simulink model "HVDCMMCInterconnection"  (R2023b)
settings: Solver=FixedStepDiscrete  StartTime=0.0  StopTime=10  FixedStep=Ts_Power  RelTol=1e-4
PreLoadFcn:
  | HVDCMMCInterconnectionParam
StartFcn:
  | tic
StopFcn:
  | toc
values from neighbouring files (symbols this model uses):
  C_PM = 1.758e-3    (= 0.001758)    [HVDCMMCInterconnectionParam.m]
  Cg = 50e-9    (= 5e-08)    [HVDCMMCInterconnectionParam.m]
  D_R = 0.001    [HVDCMMCInterconnectionParam.m]
  D_Rs = 1e8    (= 100000000)    [HVDCMMCInterconnectionParam.m]
  D_Vf = 0    [HVDCMMCInterconnectionParam.m]
  Fnom = 50    [HVDCMMCInterconnectionParam.m]
  HRM = 2    [HVDCMMCInterconnectionParam.m]
  Ki_Ireg = 6    [HVDCMMCInterconnectionParam.m]
  Ki_Preg = 1.0    (= 1)    [HVDCMMCInterconnectionParam.m]
  Ki_Qreg = 1.0    (= 1)    [HVDCMMCInterconnectionParam.m]
  Ki_VDCreg = 100    [HVDCMMCInterconnectionParam.m]
  Kp_Ireg = 0.6    [HVDCMMCInterconnectionParam.m]
  Kp_Preg = 0.5/3    (= 0.166666666667)    [HVDCMMCInterconnectionParam.m]
  Kp_Qreg = 0.5/3    (= 0.166666666667)    [HVDCMMCInterconnectionParam.m]
  Kp_VDCreg = 4    [HVDCMMCInterconnectionParam.m]
  L_cable = 15e-3    (= 0.015)    [HVDCMMCInterconnectionParam.m]
  Larm = Larm_pu*(Zb_ac/(2*pi*Fnom))    [HVDCMMCInterconnectionParam.m]
  Lff = Larm_pu/2    (= 0.075)    [HVDCMMCInterconnectionParam.m]
  Limits_Ireg = [ 2.0  -2.0]    [HVDCMMCInterconnectionParam.m]
  Limits_Preg = [ 1.2, 0.8 ]    [HVDCMMCInterconnectionParam.m]
  Limits_Qreg = [ 0.25, -0.25 ]    [HVDCMMCInterconnectionParam.m]
  Limits_VDCreg = [ 2.0  -2.0]    [HVDCMMCInterconnectionParam.m]
  Lxfo = 0.12    [HVDCMMCInterconnectionParam.m]
  Nb_PM = 36    [HVDCMMCInterconnectionParam.m]
  Pnom = 1000e6    (= 1000000000)    [HVDCMMCInterconnectionParam.m]
  R_cable = 0.5    [HVDCMMCInterconnectionParam.m]
  R_startup = 400    [HVDCMMCInterconnectionParam.m]
  Rarm = Rarm_pu*Zb_ac    [HVDCMMCInterconnectionParam.m]
  Rff = Rarm_pu/2    (= 0.00075)    [HVDCMMCInterconnectionParam.m]
  Rg = 100    [HVDCMMCInterconnectionParam.m]
  Rxfo = 0.003    [HVDCMMCInterconnectionParam.m]
  Slope_Pref = 0.5    [HVDCMMCInterconnectionParam.m]
  Slope_Qref = 0.5    [HVDCMMCInterconnectionParam.m]
  Slope_Vdc_ref = Vnom_dc/5    (= 128000)    [HVDCMMCInterconnectionParam.m]
  Tbrk1_On = 0.1    [HVDCMMCInterconnectionParam.m]
  Tbrk2_On = 1.0    (= 1)    [HVDCMMCInterconnectionParam.m]
  Tdeblock = 1.5    [HVDCMMCInterconnectionParam.m]
  Tfault = 9999    [HVDCMMCInterconnectionParam.m]
  Ton_Converter2 = 4    [HVDCMMCInterconnectionParam.m]
  Ton_PQreg = 4    [HVDCMMCInterconnectionParam.m]
  Ton_VDCreg = 1.5    [HVDCMMCInterconnectionParam.m]
  Ts = Ts_Control    (= 4e-05)    [HVDCMMCInterconnectionParam.m]    (also in power_circ2ss_sps_calc.m = 1e-06)
  Ts_Control = 40e-6    (= 4e-05)    [HVDCMMCInterconnectionParam.m]
  Ts_Power = 20e-6    (= 2e-05)    [HVDCMMCInterconnectionParam.m]
  Vb_ac = sqrt(2/3)*Vnom_sec    [HVDCMMCInterconnectionParam.m]
  Vb_dc = Vnom_dc    (= 640000)    [HVDCMMCInterconnectionParam.m]
  Vc0_PM = 0    [HVDCMMCInterconnectionParam.m]
  Vnom_dc = 640e3    (= 640000)    [HVDCMMCInterconnectionParam.m]
  Vnom_prim = 400e3    (= 400000)    [HVDCMMCInterconnectionParam.m]
  Vnom_sec = 333e3    (= 333000)    [HVDCMMCInterconnectionParam.m]
  w = 2*pi*Fnom    (= 314.159265359)    [HVDCMMCInterconnectionParam.m]
undefined symbols (not defined in the file or in its folder): ACDC, ACDC3, DiscIntNeverNeededParam, gcbh, Pcc, S, sps_AC, sps_rtmsupport
libraries: simulink x61, spsControlledVoltageSourceLib x56, spsCurrentMeasurementLib x56, spsDiodeLib x40, spsSeriesRLCBranchLib x32, spsVoltageMeasurementLib x20, powerlib_extras x9, spsHalfBridgeMMCmodel x8, spsGroundLib x7, spsSecondOrderFilterLib x6, spsabctodq0Lib x6, spsMeanLib x3
(part 4 of 11)

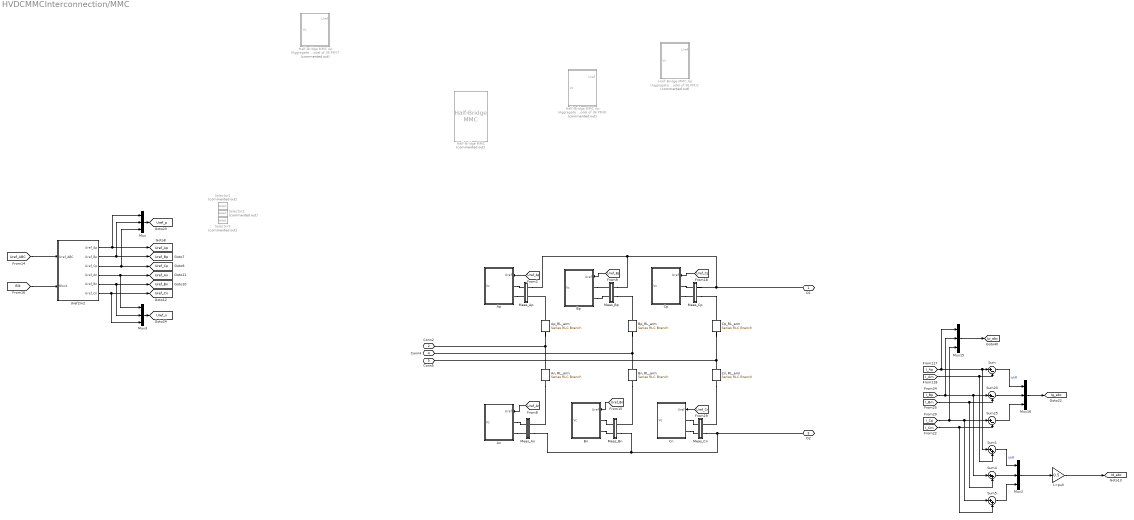
== system HVDCMMCInterconnection/MMC ==
  An : Subsystem  DialogController=POWERSYS.PowerSysDialog  LoadFcn=sps_rtmsupport('LoadFcn',gcbh);  StartFcn=sps_rtmsupport('StartFcn',gcbh);  StopFcn=sps_rtmsupport('StopFcn',gcbh);  mask(Half-Bridge MMC){ModelType=Aggregate model, n=36, C=C_PM, Vc_Initial=Vc0_PM, Ron=1e-3, Rs=1e6, Cs=inf, Ron_Diode=1e-3, Rs_Diode=1e6, Cs_Diode=inf, Vf_Diode=1e-3, Rs_CurrentSource=inf, Ts=Ts_Power}
      mask prompts: ModelType "Model type:"; n "Number of power modules"; C "Capacitor value (F)"; Vc_Initial "Capacitor initial voltage (V):"; Ron "Device on-state resistance (Ohms)"; Rs "Snubber resistance (Ohms)"; Cs "Snubber capacitance (F)"; Ron_Diode "Diode on-state resistance (Ohms)"; Rs_Diode "Diode snubber resistance (Ohms)"; Cs_Diode "Diode snubber capacitance (F)"; Vf_Diode "Diode forward voltage (V)"; Rs_CurrentSource "Current source snubber resistance (Ohms)"; Ts "Sample time (s):"
      mask help: Implements a half-bridge modular multilevel converter. The converter consists of multiple series-connected power modules. Each power module consists of one half-bridge and one capacitor on the DC side.
      mask init:
      | % block=gcb;
      | % [WantBlockChoice,Index1,MT,SPID] = powericon('FullBridgeMMCInit', block, ModelType, n, Ts, 2);
      | % powericon('SetInternalModels','set',block,WantBlockChoice);
      settings: LibrarySourceBlock=spsHalfBridgeMMCLib/Half-Bridge MMC  CopyFcn=sps_rtmsupport('CopyFcn',gcbh);  DeleteFcn=sps_rtmsupport('DeleteFcn',gcbh);  UndoDeleteFcn=sps_rtmsupport('UndoDeleteFcn',gcbh);  ModelCloseFcn=sps_rtmsupport('ModelCloseFcn',gcbh);  PreSaveFcn=sps_rtmsupport('PreSaveFcn',gcbh);  PostSaveFcn=sps_rtmsupport('PostSaveFcn',gcbh);  NameChangeFcn=sps_rtmsupport('NameChangeFcn',gcbh);  PreCopyFcn=sps_rtmsupport('PreCopyFcn',gcbh);  OpenFcn=sps_rtmsupport('OpenFcn',gcbh, [1]);  CloseFcn=sps_rtmsupport('CloseFcn',gcbh);  PreDeleteFcn=sps_rtmsupport('PreDeleteFcn',gcbh);
      mask Help: helpview(psbhelp);
      mask TypeOptions ModelType: Switching devices | Switching function | Average model (Uref-controlled) | Aggregate model
      mask Callback ModelType: powericon('FullBridgeMMCCback',gcb)
      mask Display:
      | x1=-0.04;
      | plot([0.5 0.80]+x1,[0.95 0.95])
      | plot([0.5 0.5]+x1,[0.95,0.80])
      | plot([0.5 0.38]+x1,[0.80 0.74])
      | plot([0.38 0.38]+x1,[0.80 0.62])
      | plot([0.38 0.5]+x1,[0.68 0.62])
      | plot([0.5 0.5]+x1,[0.62 0.52])
      | plot([0.45 0.5 0.43]+x1,[0.68 0.62 0.60])
      | %
      | y1=0.40;
      | plot([0.5 0.5]+x1,[0.95,0.80]-y1)
      | plot([0.5 0.38]+x1,[0.80 0.74]-y1)
      | plot([0.38 0.38]+x1,[0.80 0.62]-y1)
      | plot([0.38 0.5]+x1,[0.68 0.62]-y1)
      | plot([0.5 0.5]+x1,[0.62 0.52]-y1)
      | plot([0.45 0.5 0.43]+x1,[0.68 0.62 0.60]-y1)
      | plot([0.5 0.5]+x1,[0.2,0.10])
      | plot([0.5 0.80]+x1,[0.1 0.1])
      | %
      | plot([0.5 0.6]+x1,[0.84 0.84])
      | plot([0.6 0.6]+x1,[0.84 0.74])
      | plot([0.6 0.56]+x1,[0.74 0.69])
      | plot([0.6 0.64]+x1,[0.74 0.69])
      | plot([0.56 0.64]+x1,[0.69 0.69])
      | plot([0.6 0.6]+x1,[0.69 0.57])
      | plot([0.5 0.6]+x1,[0.57 0.57])
      | plot([0.55 0.65]+x1,[0.74 0.74])
      | %
      | y2=0.4;
      | plot([0.5 0.6]+x1,[0.84 0.84]-y2)
      | plot([0.6 0.6]+x1,[0.84 0.74]-y2)
      | plot([0.6 0.56]+x1,[0.74 0.69]-y2)
      | plot([0.6 0.64]+x1,[0.74 0.69]-y2)
      | plot([0.56 0.64]+x1,[0.69 0.69]-y2)
      | plot([0.6 0.6]+x1,[0.69 0.57]-y2)
      | plot([0.5 0.6]+x1,[0.57 0.57]-y2)
      | plot([0.55 0.65]+x1,[0.74 0.74]-y2)
      | %
      | plot([0.5 0.23]+x1,[0.5 0.5])
      | plot([0.23 0.23]+x1,[0.5 0.53])
      | plot([0.23 0.23]+x1,[0.55 0.58])
      | plot([0.23 0.23]+x1,[0.61 0.64])
      | %
      | plot([0.5 0.23]+x1,[0.1 0.1])
      | plot([0.23 0.23]+x1,[0.1 0.06])
      | plot([0.23 0.23]+x1,[0.04 0.01])
      | %
      | plot([0.34 0.34]+x1,[0.65 0.75])
      | plot([0.28 0.34]+x1,[0.7 0.7])
      | %
      | plot([0.34 0.34]+x1,[0.65 0.75]-y2)
      | plot([0.28 0.34]+x1,[0.7 0.7]-y2)
      | %
      | % Capacitor
      | plot([0.8 0.8]+x1,[0.51 0.95])
      | plot([0.72 0.88]+x1,[0.51 0.51])
      | plot([0.72 0.88]+x1,[0.51 0.51]-0.04)
      | plot([0.8 0.8]+x1,[0.47 0.1])
      | 
      | color('blue')
      | % switch lower(ModelType)
      | %     case 'average model (uref-controlled)'
      | %         port_label('input',1,'Uref')
      | %     case 'aggregate model'
      | %         port_label('input',1,'Uref')
      | %     otherwise
      | %         port_label('input',1,'Uref')
      | % end
      | port_label('output',1,'m')
  An_RL_arm : spsSeriesRLCBranchLib/Series RLC Branch  LConnTagsString=__new0  RConnTagsString=__new0  BranchType=RL  Resistance=Rarm  Inductance=Larm  SetiL0=off  InitialCurrent=0  Capacitance=1e-6  Setx0=off  InitialVoltage=0  Measurements=None
  Ap : Subsystem  DialogController=POWERSYS.PowerSysDialog  LoadFcn=sps_rtmsupport('LoadFcn',gcbh);  StartFcn=sps_rtmsupport('StartFcn',gcbh);  StopFcn=sps_rtmsupport('StopFcn',gcbh);  mask(Half-Bridge MMC){ModelType=Aggregate model, n=36, C=C_PM, Vc_Initial=Vc0_PM, Ron=1e-3, Rs=1e6, Cs=inf, Ron_Diode=1e-3, Rs_Diode=1e6, Cs_Diode=inf, Vf_Diode=1e-3, Rs_CurrentSource=inf, Ts=Ts_Power}
      mask prompts: ModelType "Model type:"; n "Number of power modules"; C "Capacitor value (F)"; Vc_Initial "Capacitor initial voltage (V):"; Ron "Device on-state resistance (Ohms)"; Rs "Snubber resistance (Ohms)"; Cs "Snubber capacitance (F)"; Ron_Diode "Diode on-state resistance (Ohms)"; Rs_Diode "Diode snubber resistance (Ohms)"; Cs_Diode "Diode snubber capacitance (F)"; Vf_Diode "Diode forward voltage (V)"; Rs_CurrentSource "Current source snubber resistance (Ohms)"; Ts "Sample time (s):"
      mask help: Implements a half-bridge modular multilevel converter. The converter consists of multiple series-connected power modules. Each power module consists of one half-bridge and one capacitor on the DC side.
      mask init:
      | % block=gcb;
      | % [WantBlockChoice,Index1,MT,SPID] = powericon('FullBridgeMMCInit', block, ModelType, n, Ts, 2);
      | % powericon('SetInternalModels','set',block,WantBlockChoice);
      settings: LibrarySourceBlock=spsHalfBridgeMMCLib/Half-Bridge MMC  CopyFcn=sps_rtmsupport('CopyFcn',gcbh);  DeleteFcn=sps_rtmsupport('DeleteFcn',gcbh);  UndoDeleteFcn=sps_rtmsupport('UndoDeleteFcn',gcbh);  ModelCloseFcn=sps_rtmsupport('ModelCloseFcn',gcbh);  PreSaveFcn=sps_rtmsupport('PreSaveFcn',gcbh);  PostSaveFcn=sps_rtmsupport('PostSaveFcn',gcbh);  NameChangeFcn=sps_rtmsupport('NameChangeFcn',gcbh);  PreCopyFcn=sps_rtmsupport('PreCopyFcn',gcbh);  OpenFcn=sps_rtmsupport('OpenFcn',gcbh, [1]);  CloseFcn=sps_rtmsupport('CloseFcn',gcbh);  PreDeleteFcn=sps_rtmsupport('PreDeleteFcn',gcbh);
      mask Help: helpview(psbhelp);
      mask TypeOptions ModelType: Switching devices | Switching function | Average model (Uref-controlled) | Aggregate model
      mask Callback ModelType: powericon('FullBridgeMMCCback',gcb)
      mask Display:
      | x1=-0.04;
      | plot([0.5 0.80]+x1,[0.95 0.95])
      | plot([0.5 0.5]+x1,[0.95,0.80])
      | plot([0.5 0.38]+x1,[0.80 0.74])
      | plot([0.38 0.38]+x1,[0.80 0.62])
      | plot([0.38 0.5]+x1,[0.68 0.62])
      | plot([0.5 0.5]+x1,[0.62 0.52])
      | plot([0.45 0.5 0.43]+x1,[0.68 0.62 0.60])
      | %
      | y1=0.40;
      | plot([0.5 0.5]+x1,[0.95,0.80]-y1)
      | plot([0.5 0.38]+x1,[0.80 0.74]-y1)
      | plot([0.38 0.38]+x1,[0.80 0.62]-y1)
      | plot([0.38 0.5]+x1,[0.68 0.62]-y1)
      | plot([0.5 0.5]+x1,[0.62 0.52]-y1)
      | plot([0.45 0.5 0.43]+x1,[0.68 0.62 0.60]-y1)
      | plot([0.5 0.5]+x1,[0.2,0.10])
      | plot([0.5 0.80]+x1,[0.1 0.1])
      | %
      | plot([0.5 0.6]+x1,[0.84 0.84])
      | plot([0.6 0.6]+x1,[0.84 0.74])
      | plot([0.6 0.56]+x1,[0.74 0.69])
      | plot([0.6 0.64]+x1,[0.74 0.69])
      | plot([0.56 0.64]+x1,[0.69 0.69])
      | plot([0.6 0.6]+x1,[0.69 0.57])
      | plot([0.5 0.6]+x1,[0.57 0.57])
      | plot([0.55 0.65]+x1,[0.74 0.74])
      | %
      | y2=0.4;
      | plot([0.5 0.6]+x1,[0.84 0.84]-y2)
      | plot([0.6 0.6]+x1,[0.84 0.74]-y2)
      | plot([0.6 0.56]+x1,[0.74 0.69]-y2)
      | plot([0.6 0.64]+x1,[0.74 0.69]-y2)
      | plot([0.56 0.64]+x1,[0.69 0.69]-y2)
      | plot([0.6 0.6]+x1,[0.69 0.57]-y2)
      | plot([0.5 0.6]+x1,[0.57 0.57]-y2)
      | plot([0.55 0.65]+x1,[0.74 0.74]-y2)
      | %
      | plot([0.5 0.23]+x1,[0.5 0.5])
      | plot([0.23 0.23]+x1,[0.5 0.53])
      | plot([0.23 0.23]+x1,[0.55 0.58])
      | plot([0.23 0.23]+x1,[0.61 0.64])
      | %
      | plot([0.5 0.23]+x1,[0.1 0.1])
      | plot([0.23 0.23]+x1,[0.1 0.06])
      | plot([0.23 0.23]+x1,[0.04 0.01])
      | %
      | plot([0.34 0.34]+x1,[0.65 0.75])
      | plot([0.28 0.34]+x1,[0.7 0.7])
      | %
      | plot([0.34 0.34]+x1,[0.65 0.75]-y2)
      | plot([0.28 0.34]+x1,[0.7 0.7]-y2)
      | %
      | % Capacitor
      | plot([0.8 0.8]+x1,[0.51 0.95])
      | plot([0.72 0.88]+x1,[0.51 0.51])
      | plot([0.72 0.88]+x1,[0.51 0.51]-0.04)
      | plot([0.8 0.8]+x1,[0.47 0.1])
      | 
      | color('blue')
      | % switch lower(ModelType)
      | %     case 'average model (uref-controlled)'
      | %         port_label('input',1,'Uref')
      | %     case 'aggregate model'
      | %         port_label('input',1,'Uref')
      | %     otherwise
      | %         port_label('input',1,'Uref')
      | % end
      | port_label('output',1,'m')
  Ap_RL_arm : spsSeriesRLCBranchLib/Series RLC Branch  LConnTagsString=__new0  RConnTagsString=__new0  BranchType=RL  Resistance=Rarm  Inductance=Larm  SetiL0=off  InitialCurrent=0  Capacitance=1e-6  Setx0=off  InitialVoltage=0  Measurements=None
  Bn : Subsystem  DialogController=POWERSYS.PowerSysDialog  LoadFcn=sps_rtmsupport('LoadFcn',gcbh);  StartFcn=sps_rtmsupport('StartFcn',gcbh);  StopFcn=sps_rtmsupport('StopFcn',gcbh);  mask(Half-Bridge MMC){ModelType=Aggregate model, n=36, C=C_PM, Vc_Initial=Vc0_PM, Ron=1e-3, Rs=1e6, Cs=inf, Ron_Diode=1e-3, Rs_Diode=1e6, Cs_Diode=inf, Vf_Diode=1e-3, Rs_CurrentSource=inf, Ts=Ts_Power}
      mask prompts: ModelType "Model type:"; n "Number of power modules"; C "Capacitor value (F)"; Vc_Initial "Capacitor initial voltage (V):"; Ron "Device on-state resistance (Ohms)"; Rs "Snubber resistance (Ohms)"; Cs "Snubber capacitance (F)"; Ron_Diode "Diode on-state resistance (Ohms)"; Rs_Diode "Diode snubber resistance (Ohms)"; Cs_Diode "Diode snubber capacitance (F)"; Vf_Diode "Diode forward voltage (V)"; Rs_CurrentSource "Current source snubber resistance (Ohms)"; Ts "Sample time (s):"
      mask help: Implements a half-bridge modular multilevel converter. The converter consists of multiple series-connected power modules. Each power module consists of one half-bridge and one capacitor on the DC side.
      mask init:
      | % block=gcb;
      | % [WantBlockChoice,Index1,MT,SPID] = powericon('FullBridgeMMCInit', block, ModelType, n, Ts, 2);
      | % powericon('SetInternalModels','set',block,WantBlockChoice);
      settings: LibrarySourceBlock=spsHalfBridgeMMCLib/Half-Bridge MMC  CopyFcn=sps_rtmsupport('CopyFcn',gcbh);  DeleteFcn=sps_rtmsupport('DeleteFcn',gcbh);  UndoDeleteFcn=sps_rtmsupport('UndoDeleteFcn',gcbh);  ModelCloseFcn=sps_rtmsupport('ModelCloseFcn',gcbh);  PreSaveFcn=sps_rtmsupport('PreSaveFcn',gcbh);  PostSaveFcn=sps_rtmsupport('PostSaveFcn',gcbh);  NameChangeFcn=sps_rtmsupport('NameChangeFcn',gcbh);  PreCopyFcn=sps_rtmsupport('PreCopyFcn',gcbh);  OpenFcn=sps_rtmsupport('OpenFcn',gcbh, [1]);  CloseFcn=sps_rtmsupport('CloseFcn',gcbh);  PreDeleteFcn=sps_rtmsupport('PreDeleteFcn',gcbh);
      mask Help: helpview(psbhelp);
      mask TypeOptions ModelType: Switching devices | Switching function | Average model (Uref-controlled) | Aggregate model
      mask Callback ModelType: powericon('FullBridgeMMCCback',gcb)
      mask Display:
      | x1=-0.04;
      | plot([0.5 0.80]+x1,[0.95 0.95])
      | plot([0.5 0.5]+x1,[0.95,0.80])
      | plot([0.5 0.38]+x1,[0.80 0.74])
      | plot([0.38 0.38]+x1,[0.80 0.62])
      | plot([0.38 0.5]+x1,[0.68 0.62])
      | plot([0.5 0.5]+x1,[0.62 0.52])
      | plot([0.45 0.5 0.43]+x1,[0.68 0.62 0.60])
      | %
      | y1=0.40;
      | plot([0.5 0.5]+x1,[0.95,0.80]-y1)
      | plot([0.5 0.38]+x1,[0.80 0.74]-y1)
      | plot([0.38 0.38]+x1,[0.80 0.62]-y1)
      | plot([0.38 0.5]+x1,[0.68 0.62]-y1)
      | plot([0.5 0.5]+x1,[0.62 0.52]-y1)
      | plot([0.45 0.5 0.43]+x1,[0.68 0.62 0.60]-y1)
      | plot([0.5 0.5]+x1,[0.2,0.10])
      | plot([0.5 0.80]+x1,[0.1 0.1])
      | %
      | plot([0.5 0.6]+x1,[0.84 0.84])
      | plot([0.6 0.6]+x1,[0.84 0.74])
      | plot([0.6 0.56]+x1,[0.74 0.69])
      | plot([0.6 0.64]+x1,[0.74 0.69])
      | plot([0.56 0.64]+x1,[0.69 0.69])
      | plot([0.6 0.6]+x1,[0.69 0.57])
      | plot([0.5 0.6]+x1,[0.57 0.57])
      | plot([0.55 0.65]+x1,[0.74 0.74])
      | %
      | y2=0.4;
      | plot([0.5 0.6]+x1,[0.84 0.84]-y2)
      | plot([0.6 0.6]+x1,[0.84 0.74]-y2)
      | plot([0.6 0.56]+x1,[0.74 0.69]-y2)
      | plot([0.6 0.64]+x1,[0.74 0.69]-y2)
      | plot([0.56 0.64]+x1,[0.69 0.69]-y2)
      | plot([0.6 0.6]+x1,[0.69 0.57]-y2)
      | plot([0.5 0.6]+x1,[0.57 0.57]-y2)
      | plot([0.55 0.65]+x1,[0.74 0.74]-y2)
      | %
      | plot([0.5 0.23]+x1,[0.5 0.5])
      | plot([0.23 0.23]+x1,[0.5 0.53])
      | plot([0.23 0.23]+x1,[0.55 0.58])
      | plot([0.23 0.23]+x1,[0.61 0.64])
      | %
      | plot([0.5 0.23]+x1,[0.1 0.1])
      | plot([0.23 0.23]+x1,[0.1 0.06])
      | plot([0.23 0.23]+x1,[0.04 0.01])
      | %
      | plot([0.34 0.34]+x1,[0.65 0.75])
      | plot([0.28 0.34]+x1,[0.7 0.7])
      | %
      | plot([0.34 0.34]+x1,[0.65 0.75]-y2)
      | plot([0.28 0.34]+x1,[0.7 0.7]-y2)
      | %
      | % Capacitor
      | plot([0.8 0.8]+x1,[0.51 0.95])
      | plot([0.72 0.88]+x1,[0.51 0.51])
      | plot([0.72 0.88]+x1,[0.51 0.51]-0.04)
      | plot([0.8 0.8]+x1,[0.47 0.1])
      | 
      | color('blue')
      | % switch lower(ModelType)
      | %     case 'average model (uref-controlled)'
      | %         port_label('input',1,'Uref')
      | %     case 'aggregate model'
      | %         port_label('input',1,'Uref')
      | %     otherwise
      | %         port_label('input',1,'Uref')
      | % end
      | port_label('output',1,'m')
  Bn_RL_arm : spsSeriesRLCBranchLib/Series RLC Branch  LConnTagsString=__new0  RConnTagsString=__new0  BranchType=RL  Resistance=Rarm  Inductance=Larm  SetiL0=off  InitialCurrent=0  Capacitance=1e-6  Setx0=off  InitialVoltage=0  Measurements=None
  Bp : Subsystem  DialogController=POWERSYS.PowerSysDialog  LoadFcn=sps_rtmsupport('LoadFcn',gcbh);  StartFcn=sps_rtmsupport('StartFcn',gcbh);  StopFcn=sps_rtmsupport('StopFcn',gcbh);  mask(Half-Bridge MMC){ModelType=Aggregate model, n=36, C=C_PM, Vc_Initial=Vc0_PM, Ron=1e-3, Rs=1e6, Cs=inf, Ron_Diode=1e-3, Rs_Diode=1e6, Cs_Diode=inf, Vf_Diode=1e-3, Rs_CurrentSource=inf, Ts=Ts_Power}
      mask prompts: ModelType "Model type:"; n "Number of power modules"; C "Capacitor value (F)"; Vc_Initial "Capacitor initial voltage (V):"; Ron "Device on-state resistance (Ohms)"; Rs "Snubber resistance (Ohms)"; Cs "Snubber capacitance (F)"; Ron_Diode "Diode on-state resistance (Ohms)"; Rs_Diode "Diode snubber resistance (Ohms)"; Cs_Diode "Diode snubber capacitance (F)"; Vf_Diode "Diode forward voltage (V)"; Rs_CurrentSource "Current source snubber resistance (Ohms)"; Ts "Sample time (s):"
      mask help: Implements a half-bridge modular multilevel converter. The converter consists of multiple series-connected power modules. Each power module consists of one half-bridge and one capacitor on the DC side.
      mask init:
      | % block=gcb;
      | % [WantBlockChoice,Index1,MT,SPID] = powericon('FullBridgeMMCInit', block, ModelType, n, Ts, 2);
      | % powericon('SetInternalModels','set',block,WantBlockChoice);
      settings: LibrarySourceBlock=spsHalfBridgeMMCLib/Half-Bridge MMC  CopyFcn=sps_rtmsupport('CopyFcn',gcbh);  DeleteFcn=sps_rtmsupport('DeleteFcn',gcbh);  UndoDeleteFcn=sps_rtmsupport('UndoDeleteFcn',gcbh);  ModelCloseFcn=sps_rtmsupport('ModelCloseFcn',gcbh);  PreSaveFcn=sps_rtmsupport('PreSaveFcn',gcbh);  PostSaveFcn=sps_rtmsupport('PostSaveFcn',gcbh);  NameChangeFcn=sps_rtmsupport('NameChangeFcn',gcbh);  PreCopyFcn=sps_rtmsupport('PreCopyFcn',gcbh);  OpenFcn=sps_rtmsupport('OpenFcn',gcbh, [1]);  CloseFcn=sps_rtmsupport('CloseFcn',gcbh);  PreDeleteFcn=sps_rtmsupport('PreDeleteFcn',gcbh);
      mask Help: helpview(psbhelp);
      mask TypeOptions ModelType: Switching devices | Switching function | Average model (Uref-controlled) | Aggregate model
      mask Callback ModelType: powericon('FullBridgeMMCCback',gcb)
      mask Display:
      | x1=-0.04;
      | plot([0.5 0.80]+x1,[0.95 0.95])
      | plot([0.5 0.5]+x1,[0.95,0.80])
      | plot([0.5 0.38]+x1,[0.80 0.74])
      | plot([0.38 0.38]+x1,[0.80 0.62])
      | plot([0.38 0.5]+x1,[0.68 0.62])
      | plot([0.5 0.5]+x1,[0.62 0.52])
      | plot([0.45 0.5 0.43]+x1,[0.68 0.62 0.60])
      | %
      | y1=0.40;
      | plot([0.5 0.5]+x1,[0.95,0.80]-y1)
      | plot([0.5 0.38]+x1,[0.80 0.74]-y1)
      | plot([0.38 0.38]+x1,[0.80 0.62]-y1)
      | plot([0.38 0.5]+x1,[0.68 0.62]-y1)
      | plot([0.5 0.5]+x1,[0.62 0.52]-y1)
      | plot([0.45 0.5 0.43]+x1,[0.68 0.62 0.60]-y1)
      | plot([0.5 0.5]+x1,[0.2,0.10])
      | plot([0.5 0.80]+x1,[0.1 0.1])
      | %
      | plot([0.5 0.6]+x1,[0.84 0.84])
      | plot([0.6 0.6]+x1,[0.84 0.74])
      | plot([0.6 0.56]+x1,[0.74 0.69])
      | plot([0.6 0.64]+x1,[0.74 0.69])
      | plot([0.56 0.64]+x1,[0.69 0.69])
      | plot([0.6 0.6]+x1,[0.69 0.57])
      | plot([0.5 0.6]+x1,[0.57 0.57])
      | plot([0.55 0.65]+x1,[0.74 0.74])
      | %
      | y2=0.4;
      | plot([0.5 0.6]+x1,[0.84 0.84]-y2)
      | plot([0.6 0.6]+x1,[0.84 0.74]-y2)
      | plot([0.6 0.56]+x1,[0.74 0.69]-y2)
      | plot([0.6 0.64]+x1,[0.74 0.69]-y2)
      | plot([0.56 0.64]+x1,[0.69 0.69]-y2)
      | plot([0.6 0.6]+x1,[0.69 0.57]-y2)
      | plot([0.5 0.6]+x1,[0.57 0.57]-y2)
      | plot([0.55 0.65]+x1,[0.74 0.74]-y2)
      | %
      | plot([0.5 0.23]+x1,[0.5 0.5])
      | plot([0.23 0.23]+x1,[0.5 0.53])
      | plot([0.23 0.23]+x1,[0.55 0.58])
      | plot([0.23 0.23]+x1,[0.61 0.64])
      | %
      | plot([0.5 0.23]+x1,[0.1 0.1])
      | plot([0.23 0.23]+x1,[0.1 0.06])
      | plot([0.23 0.23]+x1,[0.04 0.01])
      | %
      | plot([0.34 0.34]+x1,[0.65 0.75])
      | plot([0.28 0.34]+x1,[0.7 0.7])
      | %
      | plot([0.34 0.34]+x1,[0.65 0.75]-y2)
      | plot([0.28 0.34]+x1,[0.7 0.7]-y2)
      | %
      | % Capacitor
      | plot([0.8 0.8]+x1,[0.51 0.95])
      | plot([0.72 0.88]+x1,[0.51 0.51])
      | plot([0.72 0.88]+x1,[0.51 0.51]-0.04)
      | plot([0.8 0.8]+x1,[0.47 0.1])
      | 
      | color('blue')
      | % switch lower(ModelType)
      | %     case 'average model (uref-controlled)'
      | %         port_label('input',1,'Uref')
      | %     case 'aggregate model'
      | %         port_label('input',1,'Uref')
      | %     otherwise
      | %         port_label('input',1,'Uref')
      | % end
      | port_label('output',1,'m')
  Bp_RL_arm : spsSeriesRLCBranchLib/Series RLC Branch  LConnTagsString=__new0  RConnTagsString=__new0  BranchType=RL  Resistance=Rarm  Inductance=Larm  SetiL0=off  InitialCurrent=0  Capacitance=1e-6  Setx0=off  InitialVoltage=0  Measurements=None
  Cn : Subsystem  DialogController=POWERSYS.PowerSysDialog  LoadFcn=sps_rtmsupport('LoadFcn',gcbh);  StartFcn=sps_rtmsupport('StartFcn',gcbh);  StopFcn=sps_rtmsupport('StopFcn',gcbh);  mask(Half-Bridge MMC){ModelType=Aggregate model, n=36, C=C_PM, Vc_Initial=Vc0_PM, Ron=1e-3, Rs=1e6, Cs=inf, Ron_Diode=1e-3, Rs_Diode=1e6, Cs_Diode=inf, Vf_Diode=1e-3, Rs_CurrentSource=inf, Ts=Ts_Power}
      mask prompts: ModelType "Model type:"; n "Number of power modules"; C "Capacitor value (F)"; Vc_Initial "Capacitor initial voltage (V):"; Ron "Device on-state resistance (Ohms)"; Rs "Snubber resistance (Ohms)"; Cs "Snubber capacitance (F)"; Ron_Diode "Diode on-state resistance (Ohms)"; Rs_Diode "Diode snubber resistance (Ohms)"; Cs_Diode "Diode snubber capacitance (F)"; Vf_Diode "Diode forward voltage (V)"; Rs_CurrentSource "Current source snubber resistance (Ohms)"; Ts "Sample time (s):"
      mask help: Implements a half-bridge modular multilevel converter. The converter consists of multiple series-connected power modules. Each power module consists of one half-bridge and one capacitor on the DC side.
      mask init:
      | % block=gcb;
      | % [WantBlockChoice,Index1,MT,SPID] = powericon('FullBridgeMMCInit', block, ModelType, n, Ts, 2);
      | % powericon('SetInternalModels','set',block,WantBlockChoice);
      settings: LibrarySourceBlock=spsHalfBridgeMMCLib/Half-Bridge MMC  CopyFcn=sps_rtmsupport('CopyFcn',gcbh);  DeleteFcn=sps_rtmsupport('DeleteFcn',gcbh);  UndoDeleteFcn=sps_rtmsupport('UndoDeleteFcn',gcbh);  ModelCloseFcn=sps_rtmsupport('ModelCloseFcn',gcbh);  PreSaveFcn=sps_rtmsupport('PreSaveFcn',gcbh);  PostSaveFcn=sps_rtmsupport('PostSaveFcn',gcbh);  NameChangeFcn=sps_rtmsupport('NameChangeFcn',gcbh);  PreCopyFcn=sps_rtmsupport('PreCopyFcn',gcbh);  OpenFcn=sps_rtmsupport('OpenFcn',gcbh, [1]);  CloseFcn=sps_rtmsupport('CloseFcn',gcbh);  PreDeleteFcn=sps_rtmsupport('PreDeleteFcn',gcbh);
      mask Help: helpview(psbhelp);
      mask TypeOptions ModelType: Switching devices | Switching function | Average model (Uref-controlled) | Aggregate model
      mask Callback ModelType: powericon('FullBridgeMMCCback',gcb)
      mask Display:
      | x1=-0.04;
      | plot([0.5 0.80]+x1,[0.95 0.95])
      | plot([0.5 0.5]+x1,[0.95,0.80])
      | plot([0.5 0.38]+x1,[0.80 0.74])
      | plot([0.38 0.38]+x1,[0.80 0.62])
      | plot([0.38 0.5]+x1,[0.68 0.62])
      | plot([0.5 0.5]+x1,[0.62 0.52])
      | plot([0.45 0.5 0.43]+x1,[0.68 0.62 0.60])
      | %
      | y1=0.40;
      | plot([0.5 0.5]+x1,[0.95,0.80]-y1)
      | plot([0.5 0.38]+x1,[0.80 0.74]-y1)
      | plot([0.38 0.38]+x1,[0.80 0.62]-y1)
      | plot([0.38 0.5]+x1,[0.68 0.62]-y1)
      | plot([0.5 0.5]+x1,[0.62 0.52]-y1)
      | plot([0.45 0.5 0.43]+x1,[0.68 0.62 0.60]-y1)
      | plot([0.5 0.5]+x1,[0.2,0.10])
      | plot([0.5 0.80]+x1,[0.1 0.1])
      | %
      | plot([0.5 0.6]+x1,[0.84 0.84])
      | plot([0.6 0.6]+x1,[0.84 0.74])
      | plot([0.6 0.56]+x1,[0.74 0.69])
      | plot([0.6 0.64]+x1,[0.74 0.69])
      | plot([0.56 0.64]+x1,[0.69 0.69])
      | plot([0.6 0.6]+x1,[0.69 0.57])
      | plot([0.5 0.6]+x1,[0.57 0.57])
      | plot([0.55 0.65]+x1,[0.74 0.74])
      | %
      | y2=0.4;
      | plot([0.5 0.6]+x1,[0.84 0.84]-y2)
      | plot([0.6 0.6]+x1,[0.84 0.74]-y2)
      | plot([0.6 0.56]+x1,[0.74 0.69]-y2)
      | plot([0.6 0.64]+x1,[0.74 0.69]-y2)
      | plot([0.56 0.64]+x1,[0.69 0.69]-y2)
      | plot([0.6 0.6]+x1,[0.69 0.57]-y2)
      | plot([0.5 0.6]+x1,[0.57 0.57]-y2)
      | plot([0.55 0.65]+x1,[0.74 0.74]-y2)
      | %
      | plot([0.5 0.23]+x1,[0.5 0.5])
      | plot([0.23 0.23]+x1,[0.5 0.53])
      | plot([0.23 0.23]+x1,[0.55 0.58])
      | plot([0.23 0.23]+x1,[0.61 0.64])
      | %
      | plot([0.5 0.23]+x1,[0.1 0.1])
      | plot([0.23 0.23]+x1,[0.1 0.06])
      | plot([0.23 0.23]+x1,[0.04 0.01])
      | %
      | plot([0.34 0.34]+x1,[0.65 0.75])
      | plot([0.28 0.34]+x1,[0.7 0.7])
      | %
      | plot([0.34 0.34]+x1,[0.65 0.75]-y2)
      | plot([0.28 0.34]+x1,[0.7 0.7]-y2)
      | %
      | % Capacitor
      | plot([0.8 0.8]+x1,[0.51 0.95])
      | plot([0.72 0.88]+x1,[0.51 0.51])
      | plot([0.72 0.88]+x1,[0.51 0.51]-0.04)
      | plot([0.8 0.8]+x1,[0.47 0.1])
      | 
      | color('blue')
      | % switch lower(ModelType)
      | %     case 'average model (uref-controlled)'
      | %         port_label('input',1,'Uref')
      | %     case 'aggregate model'
      | %         port_label('input',1,'Uref')
      | %     otherwise
      | %         port_label('input',1,'Uref')
      | % end
      | port_label('output',1,'m')
  Cn_RL_arm : spsSeriesRLCBranchLib/Series RLC Branch  LConnTagsString=__new0  RConnTagsString=__new0  BranchType=RL  Resistance=Rarm  Inductance=Larm  SetiL0=off  InitialCurrent=0  Capacitance=1e-6  Setx0=off  InitialVoltage=0  Measurements=None
  Cp : Subsystem  DialogController=POWERSYS.PowerSysDialog  LoadFcn=sps_rtmsupport('LoadFcn',gcbh);  StartFcn=sps_rtmsupport('StartFcn',gcbh);  StopFcn=sps_rtmsupport('StopFcn',gcbh);  mask(Half-Bridge MMC){ModelType=Aggregate model, n=36, C=C_PM, Vc_Initial=Vc0_PM, Ron=1e-3, Rs=1e6, Cs=inf, Ron_Diode=1e-3, Rs_Diode=1e6, Cs_Diode=inf, Vf_Diode=1e-3, Rs_CurrentSource=inf, Ts=Ts_Power}
      mask prompts: ModelType "Model type:"; n "Number of power modules"; C "Capacitor value (F)"; Vc_Initial "Capacitor initial voltage (V):"; Ron "Device on-state resistance (Ohms)"; Rs "Snubber resistance (Ohms)"; Cs "Snubber capacitance (F)"; Ron_Diode "Diode on-state resistance (Ohms)"; Rs_Diode "Diode snubber resistance (Ohms)"; Cs_Diode "Diode snubber capacitance (F)"; Vf_Diode "Diode forward voltage (V)"; Rs_CurrentSource "Current source snubber resistance (Ohms)"; Ts "Sample time (s):"
      mask help: Implements a half-bridge modular multilevel converter. The converter consists of multiple series-connected power modules. Each power module consists of one half-bridge and one capacitor on the DC side.
      mask init:
      | % block=gcb;
      | % [WantBlockChoice,Index1,MT,SPID] = powericon('FullBridgeMMCInit', block, ModelType, n, Ts, 2);
      | % powericon('SetInternalModels','set',block,WantBlockChoice);
      settings: LibrarySourceBlock=spsHalfBridgeMMCLib/Half-Bridge MMC  CopyFcn=sps_rtmsupport('CopyFcn',gcbh);  DeleteFcn=sps_rtmsupport('DeleteFcn',gcbh);  UndoDeleteFcn=sps_rtmsupport('UndoDeleteFcn',gcbh);  ModelCloseFcn=sps_rtmsupport('ModelCloseFcn',gcbh);  PreSaveFcn=sps_rtmsupport('PreSaveFcn',gcbh);  PostSaveFcn=sps_rtmsupport('PostSaveFcn',gcbh);  NameChangeFcn=sps_rtmsupport('NameChangeFcn',gcbh);  PreCopyFcn=sps_rtmsupport('PreCopyFcn',gcbh);  OpenFcn=sps_rtmsupport('OpenFcn',gcbh, [1]);  CloseFcn=sps_rtmsupport('CloseFcn',gcbh);  PreDeleteFcn=sps_rtmsupport('PreDeleteFcn',gcbh);
      mask Help: helpview(psbhelp);
      mask TypeOptions ModelType: Switching devices | Switching function | Average model (Uref-controlled) | Aggregate model
      mask Callback ModelType: powericon('FullBridgeMMCCback',gcb)
      mask Display:
      | x1=-0.04;
      | plot([0.5 0.80]+x1,[0.95 0.95])
      | plot([0.5 0.5]+x1,[0.95,0.80])
      | plot([0.5 0.38]+x1,[0.80 0.74])
      | plot([0.38 0.38]+x1,[0.80 0.62])
      | plot([0.38 0.5]+x1,[0.68 0.62])
      | plot([0.5 0.5]+x1,[0.62 0.52])
      | plot([0.45 0.5 0.43]+x1,[0.68 0.62 0.60])
      | %
      | y1=0.40;
      | plot([0.5 0.5]+x1,[0.95,0.80]-y1)
      | plot([0.5 0.38]+x1,[0.80 0.74]-y1)
      | plot([0.38 0.38]+x1,[0.80 0.62]-y1)
      | plot([0.38 0.5]+x1,[0.68 0.62]-y1)
      | plot([0.5 0.5]+x1,[0.62 0.52]-y1)
      | plot([0.45 0.5 0.43]+x1,[0.68 0.62 0.60]-y1)
      | plot([0.5 0.5]+x1,[0.2,0.10])
      | plot([0.5 0.80]+x1,[0.1 0.1])
      | %
      | plot([0.5 0.6]+x1,[0.84 0.84])
      | plot([0.6 0.6]+x1,[0.84 0.74])
      | plot([0.6 0.56]+x1,[0.74 0.69])
      | plot([0.6 0.64]+x1,[0.74 0.69])
      | plot([0.56 0.64]+x1,[0.69 0.69])
      | plot([0.6 0.6]+x1,[0.69 0.57])
      | plot([0.5 0.6]+x1,[0.57 0.57])
      | plot([0.55 0.65]+x1,[0.74 0.74])
      | %
      | y2=0.4;
      | plot([0.5 0.6]+x1,[0.84 0.84]-y2)
      | plot([0.6 0.6]+x1,[0.84 0.74]-y2)
      | plot([0.6 0.56]+x1,[0.74 0.69]-y2)
      | plot([0.6 0.64]+x1,[0.74 0.69]-y2)
      | plot([0.56 0.64]+x1,[0.69 0.69]-y2)
      | plot([0.6 0.6]+x1,[0.69 0.57]-y2)
      | plot([0.5 0.6]+x1,[0.57 0.57]-y2)
      | plot([0.55 0.65]+x1,[0.74 0.74]-y2)
      | %
      | plot([0.5 0.23]+x1,[0.5 0.5])
      | plot([0.23 0.23]+x1,[0.5 0.53])
      | plot([0.23 0.23]+x1,[0.55 0.58])
      | plot([0.23 0.23]+x1,[0.61 0.64])
      | %
      | plot([0.5 0.23]+x1,[0.1 0.1])
      | plot([0.23 0.23]+x1,[0.1 0.06])
      | plot([0.23 0.23]+x1,[0.04 0.01])
      | %
      | plot([0.34 0.34]+x1,[0.65 0.75])
      | plot([0.28 0.34]+x1,[0.7 0.7])
      | %
      | plot([0.34 0.34]+x1,[0.65 0.75]-y2)
      | plot([0.28 0.34]+x1,[0.7 0.7]-y2)
      | %
      | % Capacitor
      | plot([0.8 0.8]+x1,[0.51 0.95])
      | plot([0.72 0.88]+x1,[0.51 0.51])
      | plot([0.72 0.88]+x1,[0.51 0.51]-0.04)
      | plot([0.8 0.8]+x1,[0.47 0.1])
      | 
      | color('blue')
      | % switch lower(ModelType)
      | %     case 'average model (uref-controlled)'
      | %         port_label('input',1,'Uref')
      | %     case 'aggregate model'
      | %         port_label('input',1,'Uref')
      | %     otherwise
      | %         port_label('input',1,'Uref')
      | % end
      | port_label('output',1,'m')
  Cp_RL_arm : spsSeriesRLCBranchLib/Series RLC Branch  LConnTagsString=__new0  RConnTagsString=__new0  BranchType=RL  Resistance=Rarm  Inductance=Larm  SetiL0=off  InitialCurrent=0  Capacitance=1e-6  Setx0=off  InitialVoltage=0  Measurements=None
  Half-Bridge MMC : spsHalfBridgeMMCLib/Half-Bridge MMC  Commented=on  ModelType=Average model (Uref-controlled)  n=1  C=10e-3  Vc_Initial=1000  Ron=1e-3  Rs=1e6  Cs=inf  Ron_Diode=1e-3  Rs_Diode=1e6  Cs_Diode=inf  Vf_Diode=1e-3  Rs_CurrentSource=inf  Ts=10e-6
      settings: LibrarySourceBlock=sps_lib/Power Electronics/Half-Bridge MMC
  Half-Bridge MMC Ap (Aggregate model of 36 PM)2 : Subsystem  Commented=on  DialogController=POWERSYS.PowerSysDialog  LoadFcn=sps_rtmsupport('LoadFcn',gcbh);  StartFcn=sps_rtmsupport('StartFcn',gcbh);  StopFcn=sps_rtmsupport('StopFcn',gcbh);  mask(Half-Bridge MMC){ModelType=Aggregate model, n=36, C=C_PM, Vc_Initial=Vc0_PM, Ron=1e-3, Rs=1e6, Cs=inf, Ron_Diode=1e-3, Rs_Diode=1e6, Cs_Diode=inf, Vf_Diode=1e-3, Rs_CurrentSource=inf, Ts=Ts_Power}
      mask prompts: ModelType "Model type:"; n "Number of power modules"; C "Capacitor value (F)"; Vc_Initial "Capacitor initial voltage (V):"; Ron "Device on-state resistance (Ohms)"; Rs "Snubber resistance (Ohms)"; Cs "Snubber capacitance (F)"; Ron_Diode "Diode on-state resistance (Ohms)"; Rs_Diode "Diode snubber resistance (Ohms)"; Cs_Diode "Diode snubber capacitance (F)"; Vf_Diode "Diode forward voltage (V)"; Rs_CurrentSource "Current source snubber resistance (Ohms)"; Ts "Sample time (s):"
      mask help: Implements a half-bridge modular multilevel converter. The converter consists of multiple series-connected power modules. Each power module consists of one half-bridge and one capacitor on the DC side.
      mask init:
      | % block=gcb;
      | % [WantBlockChoice,Index1,MT,SPID] = powericon('FullBridgeMMCInit', block, ModelType, n, Ts, 2);
      | % powericon('SetInternalModels','set',block,WantBlockChoice);
      settings: LibrarySourceBlock=spsHalfBridgeMMCLib/Half-Bridge MMC  CopyFcn=sps_rtmsupport('CopyFcn',gcbh);  DeleteFcn=sps_rtmsupport('DeleteFcn',gcbh);  UndoDeleteFcn=sps_rtmsupport('UndoDeleteFcn',gcbh);  ModelCloseFcn=sps_rtmsupport('ModelCloseFcn',gcbh);  PreSaveFcn=sps_rtmsupport('PreSaveFcn',gcbh);  PostSaveFcn=sps_rtmsupport('PostSaveFcn',gcbh);  NameChangeFcn=sps_rtmsupport('NameChangeFcn',gcbh);  PreCopyFcn=sps_rtmsupport('PreCopyFcn',gcbh);  OpenFcn=sps_rtmsupport('OpenFcn',gcbh, [1]);  CloseFcn=sps_rtmsupport('CloseFcn',gcbh);  PreDeleteFcn=sps_rtmsupport('PreDeleteFcn',gcbh);
      mask Help: helpview(psbhelp);
      mask TypeOptions ModelType: Switching devices | Switching function | Average model (Uref-controlled) | Aggregate model
      mask Callback ModelType: powericon('FullBridgeMMCCback',gcb)
      mask Display:
      | x1=-0.04;
      | plot([0.5 0.80]+x1,[0.95 0.95])
      | plot([0.5 0.5]+x1,[0.95,0.80])
      | plot([0.5 0.38]+x1,[0.80 0.74])
      | plot([0.38 0.38]+x1,[0.80 0.62])
      | plot([0.38 0.5]+x1,[0.68 0.62])
      | plot([0.5 0.5]+x1,[0.62 0.52])
      | plot([0.45 0.5 0.43]+x1,[0.68 0.62 0.60])
      | %
      | y1=0.40;
      | plot([0.5 0.5]+x1,[0.95,0.80]-y1)
      | plot([0.5 0.38]+x1,[0.80 0.74]-y1)
      | plot([0.38 0.38]+x1,[0.80 0.62]-y1)
      | plot([0.38 0.5]+x1,[0.68 0.62]-y1)
      | plot([0.5 0.5]+x1,[0.62 0.52]-y1)
      | plot([0.45 0.5 0.43]+x1,[0.68 0.62 0.60]-y1)
      | plot([0.5 0.5]+x1,[0.2,0.10])
      | plot([0.5 0.80]+x1,[0.1 0.1])
      | %
      | plot([0.5 0.6]+x1,[0.84 0.84])
      | plot([0.6 0.6]+x1,[0.84 0.74])
      | plot([0.6 0.56]+x1,[0.74 0.69])
      | plot([0.6 0.64]+x1,[0.74 0.69])
      | plot([0.56 0.64]+x1,[0.69 0.69])
      | plot([0.6 0.6]+x1,[0.69 0.57])
      | plot([0.5 0.6]+x1,[0.57 0.57])
      | plot([0.55 0.65]+x1,[0.74 0.74])
      | %
      | y2=0.4;
      | plot([0.5 0.6]+x1,[0.84 0.84]-y2)
      | plot([0.6 0.6]+x1,[0.84 0.74]-y2)
      | plot([0.6 0.56]+x1,[0.74 0.69]-y2)
      | plot([0.6 0.64]+x1,[0.74 0.69]-y2)
      | plot([0.56 0.64]+x1,[0.69 0.69]-y2)
      | plot([0.6 0.6]+x1,[0.69 0.57]-y2)
      | plot([0.5 0.6]+x1,[0.57 0.57]-y2)
      | plot([0.55 0.65]+x1,[0.74 0.74]-y2)
      | %
      | plot([0.5 0.23]+x1,[0.5 0.5])
      | plot([0.23 0.23]+x1,[0.5 0.53])
      | plot([0.23 0.23]+x1,[0.55 0.58])
      | plot([0.23 0.23]+x1,[0.61 0.64])
      | %
      | plot([0.5 0.23]+x1,[0.1 0.1])
      | plot([0.23 0.23]+x1,[0.1 0.06])
      | plot([0.23 0.23]+x1,[0.04 0.01])
      | %
      | plot([0.34 0.34]+x1,[0.65 0.75])
      | plot([0.28 0.34]+x1,[0.7 0.7])
      | %
      | plot([0.34 0.34]+x1,[0.65 0.75]-y2)
      | plot([0.28 0.34]+x1,[0.7 0.7]-y2)
      | %
      | % Capacitor
      | plot([0.8 0.8]+x1,[0.51 0.95])
      | plot([0.72 0.88]+x1,[0.51 0.51])
      | plot([0.72 0.88]+x1,[0.51 0.51]-0.04)
      | plot([0.8 0.8]+x1,[0.47 0.1])
      | 
      | color('blue')
      | % switch lower(ModelType)
      | %     case 'average model (uref-controlled)'
      | %         port_label('input',1,'Uref')
      | %     case 'aggregate model'
      | %         port_label('input',1,'Uref')
      | %     otherwise
      | %         port_label('input',1,'Uref')
      | % end
      | port_label('output',1,'m')
  Half-Bridge MMC Ap (Aggregate model of 36 PM)7 : Subsystem  Commented=on  DialogController=POWERSYS.PowerSysDialog  LoadFcn=sps_rtmsupport('LoadFcn',gcbh);  StartFcn=sps_rtmsupport('StartFcn',gcbh);  StopFcn=sps_rtmsupport('StopFcn',gcbh);  mask(Half-Bridge MMC){ModelType=Aggregate model, n=36, C=C_PM, Vc_Initial=Vc0_PM, Ron=1e-3, Rs=1e6, Cs=inf, Ron_Diode=1e-3, Rs_Diode=1e6, Cs_Diode=inf, Vf_Diode=1e-3, Rs_CurrentSource=inf, Ts=Ts_Power}
      mask prompts: ModelType "Model type:"; n "Number of power modules"; C "Capacitor value (F)"; Vc_Initial "Capacitor initial voltage (V):"; Ron "Device on-state resistance (Ohms)"; Rs "Snubber resistance (Ohms)"; Cs "Snubber capacitance (F)"; Ron_Diode "Diode on-state resistance (Ohms)"; Rs_Diode "Diode snubber resistance (Ohms)"; Cs_Diode "Diode snubber capacitance (F)"; Vf_Diode "Diode forward voltage (V)"; Rs_CurrentSource "Current source snubber resistance (Ohms)"; Ts "Sample time (s):"
      mask help: Implements a half-bridge modular multilevel converter. The converter consists of multiple series-connected power modules. Each power module consists of one half-bridge and one capacitor on the DC side.
      mask init:
      | % block=gcb;
      | % [WantBlockChoice,Index1,MT,SPID] = powericon('FullBridgeMMCInit', block, ModelType, n, Ts, 2);
      | % powericon('SetInternalModels','set',block,WantBlockChoice);
      settings: LibrarySourceBlock=spsHalfBridgeMMCLib/Half-Bridge MMC  CopyFcn=sps_rtmsupport('CopyFcn',gcbh);  DeleteFcn=sps_rtmsupport('DeleteFcn',gcbh);  UndoDeleteFcn=sps_rtmsupport('UndoDeleteFcn',gcbh);  ModelCloseFcn=sps_rtmsupport('ModelCloseFcn',gcbh);  PreSaveFcn=sps_rtmsupport('PreSaveFcn',gcbh);  PostSaveFcn=sps_rtmsupport('PostSaveFcn',gcbh);  NameChangeFcn=sps_rtmsupport('NameChangeFcn',gcbh);  PreCopyFcn=sps_rtmsupport('PreCopyFcn',gcbh);  OpenFcn=sps_rtmsupport('OpenFcn',gcbh, [1]);  CloseFcn=sps_rtmsupport('CloseFcn',gcbh);  PreDeleteFcn=sps_rtmsupport('PreDeleteFcn',gcbh);
      mask Help: helpview(psbhelp);
      mask TypeOptions ModelType: Switching devices | Switching function | Average model (Uref-controlled) | Aggregate model
      mask Callback ModelType: powericon('FullBridgeMMCCback',gcb)
      mask Display:
      | x1=-0.04;
      | plot([0.5 0.80]+x1,[0.95 0.95])
      | plot([0.5 0.5]+x1,[0.95,0.80])
      | plot([0.5 0.38]+x1,[0.80 0.74])
      | plot([0.38 0.38]+x1,[0.80 0.62])
      | plot([0.38 0.5]+x1,[0.68 0.62])
      | plot([0.5 0.5]+x1,[0.62 0.52])
      | plot([0.45 0.5 0.43]+x1,[0.68 0.62 0.60])
      | %
      | y1=0.40;
      | plot([0.5 0.5]+x1,[0.95,0.80]-y1)
      | plot([0.5 0.38]+x1,[0.80 0.74]-y1)
      | plot([0.38 0.38]+x1,[0.80 0.62]-y1)
      | plot([0.38 0.5]+x1,[0.68 0.62]-y1)
      | plot([0.5 0.5]+x1,[0.62 0.52]-y1)
      | plot([0.45 0.5 0.43]+x1,[0.68 0.62 0.60]-y1)
      | plot([0.5 0.5]+x1,[0.2,0.10])
      | plot([0.5 0.80]+x1,[0.1 0.1])
      | %
      | plot([0.5 0.6]+x1,[0.84 0.84])
      | plot([0.6 0.6]+x1,[0.84 0.74])
      | plot([0.6 0.56]+x1,[0.74 0.69])
      | plot([0.6 0.64]+x1,[0.74 0.69])
      | plot([0.56 0.64]+x1,[0.69 0.69])
      | plot([0.6 0.6]+x1,[0.69 0.57])
      | plot([0.5 0.6]+x1,[0.57 0.57])
      | plot([0.55 0.65]+x1,[0.74 0.74])
      | %
      | y2=0.4;
      | plot([0.5 0.6]+x1,[0.84 0.84]-y2)
      | plot([0.6 0.6]+x1,[0.84 0.74]-y2)
      | plot([0.6 0.56]+x1,[0.74 0.69]-y2)
      | plot([0.6 0.64]+x1,[0.74 0.69]-y2)
      | plot([0.56 0.64]+x1,[0.69 0.69]-y2)
      | plot([0.6 0.6]+x1,[0.69 0.57]-y2)
      | plot([0.5 0.6]+x1,[0.57 0.57]-y2)
      | plot([0.55 0.65]+x1,[0.74 0.74]-y2)
      | %
      | plot([0.5 0.23]+x1,[0.5 0.5])
      | plot([0.23 0.23]+x1,[0.5 0.53])
      | plot([0.23 0.23]+x1,[0.55 0.58])
      | plot([0.23 0.23]+x1,[0.61 0.64])
      | %
      | plot([0.5 0.23]+x1,[0.1 0.1])
      | plot([0.23 0.23]+x1,[0.1 0.06])
      | plot([0.23 0.23]+x1,[0.04 0.01])
      | %
      | plot([0.34 0.34]+x1,[0.65 0.75])
      | plot([0.28 0.34]+x1,[0.7 0.7])
      | %
      | plot([0.34 0.34]+x1,[0.65 0.75]-y2)
      | plot([0.28 0.34]+x1,[0.7 0.7]-y2)
      | %
      | % Capacitor
      | plot([0.8 0.8]+x1,[0.51 0.95])
      | plot([0.72 0.88]+x1,[0.51 0.51])
      | plot([0.72 0.88]+x1,[0.51 0.51]-0.04)
      | plot([0.8 0.8]+x1,[0.47 0.1])
      | 
      | color('blue')
      | % switch lower(ModelType)
      | %     case 'average model (uref-controlled)'
      | %         port_label('input',1,'Uref')
      | %     case 'aggregate model'
      | %         port_label('input',1,'Uref')
      | %     otherwise
      | %         port_label('input',1,'Uref')
      | % end
      | port_label('output',1,'m')
  Half-Bridge MMC Ap (Aggregate model of 36 PM)8 : Subsystem  Commented=on  DialogController=POWERSYS.PowerSysDialog  LoadFcn=sps_rtmsupport('LoadFcn',gcbh);  StartFcn=sps_rtmsupport('StartFcn',gcbh);  StopFcn=sps_rtmsupport('StopFcn',gcbh);  mask(Half-Bridge MMC){ModelType=Aggregate model, n=36, C=C_PM, Vc_Initial=Vc0_PM, Ron=1e-3, Rs=1e6, Cs=inf, Ron_Diode=1e-3, Rs_Diode=1e6, Cs_Diode=inf, Vf_Diode=1e-3, Rs_CurrentSource=inf, Ts=Ts_Power}
      mask prompts: ModelType "Model type:"; n "Number of power modules"; C "Capacitor value (F)"; Vc_Initial "Capacitor initial voltage (V):"; Ron "Device on-state resistance (Ohms)"; Rs "Snubber resistance (Ohms)"; Cs "Snubber capacitance (F)"; Ron_Diode "Diode on-state resistance (Ohms)"; Rs_Diode "Diode snubber resistance (Ohms)"; Cs_Diode "Diode snubber capacitance (F)"; Vf_Diode "Diode forward voltage (V)"; Rs_CurrentSource "Current source snubber resistance (Ohms)"; Ts "Sample time (s):"
      mask help: Implements a half-bridge modular multilevel converter. The converter consists of multiple series-connected power modules. Each power module consists of one half-bridge and one capacitor on the DC side.
      mask init:
      | % block=gcb;
      | % [WantBlockChoice,Index1,MT,SPID] = powericon('FullBridgeMMCInit', block, ModelType, n, Ts, 2);
      | % powericon('SetInternalModels','set',block,WantBlockChoice);
      settings: LibrarySourceBlock=spsHalfBridgeMMCLib/Half-Bridge MMC  CopyFcn=sps_rtmsupport('CopyFcn',gcbh);  DeleteFcn=sps_rtmsupport('DeleteFcn',gcbh);  UndoDeleteFcn=sps_rtmsupport('UndoDeleteFcn',gcbh);  ModelCloseFcn=sps_rtmsupport('ModelCloseFcn',gcbh);  PreSaveFcn=sps_rtmsupport('PreSaveFcn',gcbh);  PostSaveFcn=sps_rtmsupport('PostSaveFcn',gcbh);  NameChangeFcn=sps_rtmsupport('NameChangeFcn',gcbh);  PreCopyFcn=sps_rtmsupport('PreCopyFcn',gcbh);  OpenFcn=sps_rtmsupport('OpenFcn',gcbh, [1]);  CloseFcn=sps_rtmsupport('CloseFcn',gcbh);  PreDeleteFcn=sps_rtmsupport('PreDeleteFcn',gcbh);
      mask Help: helpview(psbhelp);
      mask TypeOptions ModelType: Switching devices | Switching function | Average model (Uref-controlled) | Aggregate model
      mask Callback ModelType: powericon('FullBridgeMMCCback',gcb)
      mask Display:
      | x1=-0.04;
      | plot([0.5 0.80]+x1,[0.95 0.95])
      | plot([0.5 0.5]+x1,[0.95,0.80])
      | plot([0.5 0.38]+x1,[0.80 0.74])
      | plot([0.38 0.38]+x1,[0.80 0.62])
      | plot([0.38 0.5]+x1,[0.68 0.62])
      | plot([0.5 0.5]+x1,[0.62 0.52])
      | plot([0.45 0.5 0.43]+x1,[0.68 0.62 0.60])
      | %
      | y1=0.40;
      | plot([0.5 0.5]+x1,[0.95,0.80]-y1)
      | plot([0.5 0.38]+x1,[0.80 0.74]-y1)
      | plot([0.38 0.38]+x1,[0.80 0.62]-y1)
      | plot([0.38 0.5]+x1,[0.68 0.62]-y1)
      | plot([0.5 0.5]+x1,[0.62 0.52]-y1)
      | plot([0.45 0.5 0.43]+x1,[0.68 0.62 0.60]-y1)
      | plot([0.5 0.5]+x1,[0.2,0.10])
      | plot([0.5 0.80]+x1,[0.1 0.1])
      | %
      | plot([0.5 0.6]+x1,[0.84 0.84])
      | plot([0.6 0.6]+x1,[0.84 0.74])
      | plot([0.6 0.56]+x1,[0.74 0.69])
      | plot([0.6 0.64]+x1,[0.74 0.69])
      | plot([0.56 0.64]+x1,[0.69 0.69])
      | plot([0.6 0.6]+x1,[0.69 0.57])
      | plot([0.5 0.6]+x1,[0.57 0.57])
      | plot([0.55 0.65]+x1,[0.74 0.74])
      | %
      | y2=0.4;
      | plot([0.5 0.6]+x1,[0.84 0.84]-y2)
      | plot([0.6 0.6]+x1,[0.84 0.74]-y2)
      | plot([0.6 0.56]+x1,[0.74 0.69]-y2)
      | plot([0.6 0.64]+x1,[0.74 0.69]-y2)
      | plot([0.56 0.64]+x1,[0.69 0.69]-y2)
      | plot([0.6 0.6]+x1,[0.69 0.57]-y2)
      | plot([0.5 0.6]+x1,[0.57 0.57]-y2)
      | plot([0.55 0.65]+x1,[0.74 0.74]-y2)
      | %
      | plot([0.5 0.23]+x1,[0.5 0.5])
      | plot([0.23 0.23]+x1,[0.5 0.53])
      | plot([0.23 0.23]+x1,[0.55 0.58])
      | plot([0.23 0.23]+x1,[0.61 0.64])
      | %
      | plot([0.5 0.23]+x1,[0.1 0.1])
      | plot([0.23 0.23]+x1,[0.1 0.06])
      | plot([0.23 0.23]+x1,[0.04 0.01])
      | %
      | plot([0.34 0.34]+x1,[0.65 0.75])
      | plot([0.28 0.34]+x1,[0.7 0.7])
      | %
      | plot([0.34 0.34]+x1,[0.65 0.75]-y2)
      | plot([0.28 0.34]+x1,[0.7 0.7]-y2)
      | %
      | % Capacitor
      | plot([0.8 0.8]+x1,[0.51 0.95])
      | plot([0.72 0.88]+x1,[0.51 0.51])
      | plot([0.72 0.88]+x1,[0.51 0.51]-0.04)
      | plot([0.8 0.8]+x1,[0.47 0.1])
      | 
      | color('blue')
      | % switch lower(ModelType)
      | %     case 'average model (uref-controlled)'
      | %         port_label('input',1,'Uref')
      | %     case 'aggregate model'
      | %         port_label('input',1,'Uref')
      | %     otherwise
      | %         port_label('input',1,'Uref')
      | % end
      | port_label('output',1,'m')
  I->pu3 : Gain  Gain=0.5  SaturateOnIntegerOverflow=on  OutDataTypeStr=Inherit: Same as input  ParamDataTypeStr=Inherit: Same as input
  Meas_An : Subsystem
  Meas_Ap : Subsystem
  Meas_Bn : Subsystem
  Meas_Bp : Subsystem
  Meas_Cn : Subsystem
  Meas_Cp : Subsystem
  Mux{,2..3,15..16} (5 alike) : Mux  Inputs=3
  Selector1 : Selector  Commented=on  InputPortWidth=2  IndexOptions=Index vector (dialog)  Indices=1  OutputSizes=1
  Selector2 : Selector  Commented=on  InputPortWidth=2  IndexOptions=Index vector (dialog)  Indices=1  OutputSizes=1
  Selector3 : Selector  Commented=on  InputPortWidth=2  IndexOptions=Index vector (dialog)  Indices=1  OutputSizes=1
  Sum : Sum  Inputs=|+-
  Sum1 : Sum  Inputs=|++
  Sum23 : Sum  Inputs=|+-
  Sum25 : Sum  Inputs=|+-
  Sum4 : Sum  Inputs=|++
  Sum5 : Sum  Inputs=|++
  Uref2m2 : Subsystem
  O1 : PMIOPort  Side=Right
  Conn2 : PMIOPort  Port=2  Side=Left
  O2 : PMIOPort  Port=3  Side=Right
  Conn4 : PMIOPort  Port=4  Side=Left
  Conn5 : PMIOPort  Port=5  Side=Left
  tag scope: Id_abc=global, Ig_abc=global, Ip_abc=global, Uref_An=global, Uref_Ap=global, Uref_Bn=global, Uref_Bp=global, Uref_Cn=global, Uref_Cp=global, Uref_n=global, Uref_p=global
  wires:
  [Uref_An] -> An/1(Uref)
  [Uref_Cp] -> Cp/1(Uref)
  [Uref_Cn] -> Cn/1(Uref)
  [Uref_Bp] -> Bp/1(Uref)
  Sum4/1 -> Mux2/2
  [I_Ap] -> Mux15/1, Sum1/1, Sum/1
  [I_Am] -> Sum1/2, Sum/2
  Sum25/1 -> Mux16/3
  [I_Bp] -> Mux15/2, Sum4/1, Sum23/1
  Mux15/1 -> [Ip_abc]
  [I_Bm] -> Sum4/2, Sum23/2
  Sum1/1 -> Mux2/1  "Idiff"
  Sum/1 -> Mux16/1  "Idiff"
  [I_Cm] -> Sum5/2, Sum25/2
  Sum23/1 -> Mux16/2
  [I_Cp] -> Mux15/3, Sum5/1, Sum25/1
  Sum5/1 -> Mux2/3
  Mux3/1 -> [Uref_n]
  Uref2m2/5(Uref_Bn) -> Mux3/2, [Uref_Bn]
  Uref2m2/6(Uref_Cn) -> Mux3/3, [Uref_Cn]
  Uref2m2/3(Uref_Cp) -> Mux/3, [Uref_Cp]
  Uref2m2/4(Uref_An) -> Mux3/1, [Uref_An]
  Mux/1 -> [Uref_p]
  [Uref_ABC] -> Uref2m2/1(Uref_ABC)
  [Blk] -> Uref2m2/2(Block)
  Uref2m2/1(Uref_Ap) -> Mux/1, [Uref_Ap]
  Uref2m2/2(Uref_Bp) -> Mux/2, [Uref_Bp]
  [Uref_Bn] -> Bn/1(Uref)
  [Uref_Ap] -> Ap/1(Uref)
  I->pu3/1 -> [Id_abc]
  Mux2/1 -> I->pu3/1
  Mux16/1 -> [Ig_abc]
  connections:
  An/LConn1 -- Meas_An/LConn1
  An/LConn2 -- Meas_An/LConn2
  Cp/LConn2 -- Meas_Cp/LConn2
  Meas_Ap/RConn1 -- Meas_Cp/RConn1 -- O1/RConn1 -- Meas_Bp/RConn1
  Cn/LConn1 -- Meas_Cn/LConn1
  Bp/LConn2 -- Meas_Bp/LConn2
  Bn/LConn2 -- Meas_Bn/LConn2
  Cn/LConn2 -- Meas_Cn/LConn2
  Ap_RL_arm/LConn1 -- Meas_Ap/RConn2
  Meas_An/RConn2 -- Meas_Cn/RConn2 -- O2/RConn1 -- Meas_Bn/RConn2
  Bn/LConn1 -- Meas_Bn/LConn1
  Conn2/RConn1 -- Ap_RL_arm/RConn1 -- An_RL_arm/LConn1
  Ap/LConn1 -- Meas_Ap/LConn1
  Conn4/RConn1 -- Bp_RL_arm/RConn1 -- Bn_RL_arm/LConn1
  Bp/LConn1 -- Meas_Bp/LConn1
  Cp/LConn1 -- Meas_Cp/LConn1
  Conn5/RConn1 -- Cp_RL_arm/RConn1 -- Cn_RL_arm/LConn1
  Ap/LConn2 -- Meas_Ap/LConn2
  Meas_Bp/RConn2 -- Bp_RL_arm/LConn1
  Meas_Cp/RConn2 -- Cp_RL_arm/LConn1
  An_RL_arm/RConn1 -- Meas_An/RConn1
  Bn_RL_arm/RConn1 -- Meas_Bn/RConn1
  Cn_RL_arm/RConn1 -- Meas_Cn/RConn1
